simulink model "raspberrypi_sensehat_autorotate"  (R2018b)
settings: Solver=FixedStepAuto  StartTime=0.0  StopTime=inf  RelTol=1e-3
libraries: sensehatlib x2
settings Model: SimulationMode=external  Creator=The MathWorks, Inc.  LastModifiedBy=The MathWorks, Inc.
settings SolverCC: PositivePriorityOrder=on
settings OptimizationCC: MaxStackSize=64
settings DebuggingCC: ParameterTunabilityLossMsg=error
settings HardwareCC: ProdBitPerPointer=32  ProdBitPerSizeT=32  ProdBitPerPtrDiffT=32  ProdLargestAtomicInteger=Long  ProdLargestAtomicFloat=Double  ProdWordSize=32  ProdHWDeviceType=ARM Compatible->ARM Cortex  UseEmbeddedCoderFeatures=off  UseSimulinkCoderFeatures=off
settings SFSimCC: SimUseLocalCustomCode=off
settings RTWCC: SystemTargetFile=ert.tlc  HardwareBoard=Raspberry Pi  TLCOptions="-aInlineSetEventsForThisBaseRateFcn=TLC_FALSE -aSuppressMultiTaskScheduler=TLC_FALSE  -aRateBasedStepFcn=0"  TemplateMakefile=ert_default_tmf  GenerateReport=on  RTWUseLocalCustomCode=off  Toolchain=GNU GCC Raspberry Pi  LaunchReport=on
settings CodeAppCC: ForceParamTrailComments=on  OperatorAnnotations=on  StateflowObjectComments=on  MATLABSourceComments=on
settings ERTTargetCC: ERTCustomFileBanners=off  SupportContinuousTime=on  SupportNonInlinedSFcns=on  RemoveResetFunc=off  SupportVariableSizeSignals=on  ModelStepFunctionPrototypeControlCompliant=off

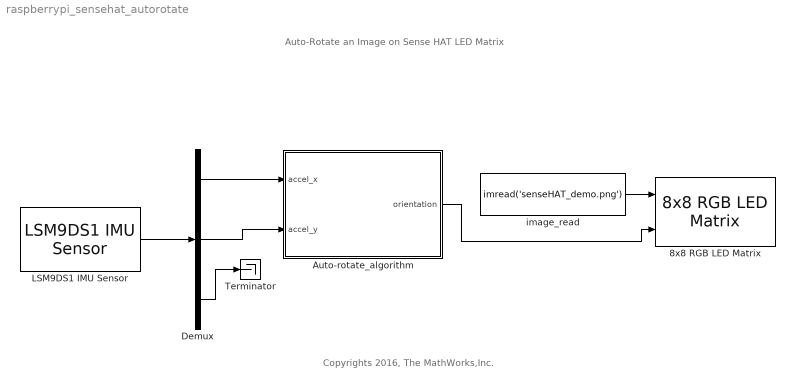
== system raspberrypi_sensehat_autorotate ==
  note: Copyrights 2016, The MathWorks,Inc.
  note: Auto-Rotate an Image
      | on
      | Sense HAT LED Matrix
  "8x8 RGB LED Matrix " : sensehatlib/8x8 RGB LED Matrix   Mode=Display Image  ImageSource=One multidimensional signal  OrientationSource=Input port  LEDOrientation=0  blockPlatform=Raspberry pi
      settings: SourceProductName=Simulink Support Package for Raspberry Pi Hardware
  "Auto-rotate_algorithm " : Stateflow chart  TreatAsAtomicUnit=on
  Demux : Demux  Outputs=3
  LSM9DS1 IMU Sensor : sensehatlib/LSM9DS1 IMU Sensor  blockPlatform=Raspberry Pi  BoardProperty_sh=Pi 2 Model B  ActiveSensors_=Accelerometer  AccelerometerOutputDataRate=119 Hz  AccelerometerFullScaleRange=+/- 2g  AccelerometerBandwidth=50 Hz  GyroscopeOutputDataRate=119 Hz  GyroscopeFullScaleRange=245 dps  GyroscopeBandwidthMode=0  GyroscopeHighPassFilterEnabled=off  GyroscopeHighPassFilterMode=0  MagnetometerFullScaleRange=+/- 4 gauss  MagnetometerOutputDataRate=40 Hz  SampleTime=0.1
      settings: SourceProductName=Simulink Support Package for Raspberry Pi Hardware
  Terminator : Terminator
  image_read : Constant  Value=imread('senseHAT_demo.png')
  wires:
  LSM9DS1 IMU Sensor/1 -> Demux/1
  Demux/1 -> "Auto-rotate_algorithm "/1(accel_x)
  Demux/2 -> "Auto-rotate_algorithm "/2(accel_y)
  Demux/3 -> Terminator/1
  "Auto-rotate_algorithm "/1(orientation) -> "8x8 RGB LED Matrix "/2
  image_read/1 -> "8x8 RGB LED Matrix "/1

== stateflow chart raspberrypi_sensehat_autorotate/Auto-rotate_algorithm  ==
  state Orientation_180
    entry:
    orientation = uint16(180);
  state Orientation_0
    entry:
    orientation=uint16(0);
  state Orientation_90
    entry:
    orientation=uint16(90);
  state Orientation_270
    entry:
    orientation = uint16(270);
  Orientation_0 -> Orientation_180 [order 3] : [accel_y >0.75]
  (default) -> Orientation_0
  Orientation_180 -> Orientation_0 [order 3] : [accel_y < -0.75]
  Orientation_180 -> Orientation_90 [order 1] : [accel_x > 0.75]
  Orientation_270 -> Orientation_0 [order 1] : [accel_y < -0.75]
  Orientation_90 -> Orientation_180 [order 2] : [accel_y >0.75]
  Orientation_0 -> Orientation_270 [order 2] : [accel_x < -0.75]
  Orientation_180 -> Orientation_270 [order 2] : [accel_x < -0.75]
  Orientation_270 -> Orientation_180 [order 2] : [accel_y >0.75]
  Orientation_0 -> Orientation_90 [order 1] : [accel_x > 0.75]
  Orientation_90 -> Orientation_0 [order 1] : [accel_y < -0.75]
  Orientation_90 -> Orientation_270 [order 3] : [accel_x < -0.75]
  Orientation_270 -> Orientation_90 [order 3] : [accel_x > 0.75]
  data: orientation output uint16; accel_x input; accel_y input
